simulink model "Battery_Connected_3_Phase_GridTied_Inverter"  (R2022a)
settings: Solver=ode3  StartTime=0.0  StopTime=4  FixedStep=dtsim  RelTol=1e-3
values from neighbouring files (symbols this model uses):
  a1_lpf = 1.3601/wc_lpf    (= 4.32933276199e-05)    [Battery_Connected_3_Phase_GridTied_Inverter_Parameters.m]    (also in NonDispDGParameters.m)
  a2_lpf = 0.6165/wc_lpf2    (= 6.24645097155e-10)    [Battery_Connected_3_Phase_GridTied_Inverter_Parameters.m]    (also in NonDispDGParameters.m)
  bf = 2 * eta * wc    [Battery_Connected_3_Phase_GridTied_Inverter_Parameters.m]    (also in NonDispDGParameters.m)
  C_HV = 100e-6    (= 0.0001)    [Battery_Connected_3_Phase_GridTied_Inverter_Parameters.m]    (also in NonDispDGParameters.m; power_converters_DAB_1ph_Parameters.m)
  C_LV = 2000e-6    (= 0.002)    [Battery_Connected_3_Phase_GridTied_Inverter_Parameters.m]    (also in NonDispDGParameters.m; power_converters_DAB_1ph_Parameters.m)
  Cdc = 2 * E_Cdc / Vdc / Vdc    (= 0.00125)    [Battery_Connected_3_Phase_GridTied_Inverter_Parameters.m]    (also in NonDispDGParameters.m)
  Cf = x*Cb    (= 7.95774715459e-06)    [Battery_Connected_3_Phase_GridTied_Inverter_Parameters.m]    (also in NonDispDGParameters.m = 8.72536076817e-06)
  cf = wc * wc    (= 15791.3670417)    [Battery_Connected_3_Phase_GridTied_Inverter_Parameters.m]    (also in NonDispDGParameters.m)
  Cs_FET = inf    [Battery_Connected_3_Phase_GridTied_Inverter_Parameters.m]    (also in NonDispDGParameters.m; power_converters_DAB_1ph_Parameters.m)
  dP1 = 0.3    [Battery_Connected_3_Phase_GridTied_Inverter_Parameters.m]    (also in NonDispDGParameters.m)
  dP2 = 0.5    [Battery_Connected_3_Phase_GridTied_Inverter_Parameters.m]    (also in NonDispDGParameters.m)
  dP3 = 0.8    [Battery_Connected_3_Phase_GridTied_Inverter_Parameters.m]    (also in NonDispDGParameters.m = 0.2)
  dP4 = -0.6    [Battery_Connected_3_Phase_GridTied_Inverter_Parameters.m]    (also in NonDispDGParameters.m)
  dtsim = 5.0e-6    (= 5e-06)    [Battery_Connected_3_Phase_GridTied_Inverter_Parameters.m]    (also in NonDispDGParameters.m)
  f0 = 50    [Battery_Connected_3_Phase_GridTied_Inverter_Parameters.m]    (also in NonDispDGParameters.m)
  Fsw = 10e3    (= 10000)    [Battery_Connected_3_Phase_GridTied_Inverter_Parameters.m]    (also in NonDispDGParameters.m; power_converters_DAB_1ph_Parameters.m = 5000)
  Ia_limit = 1    [Battery_Connected_3_Phase_GridTied_Inverter_Parameters.m]    (also in NonDispDGParameters.m)
  Ib_peak = Ib*sqrt(2)    [Battery_Connected_3_Phase_GridTied_Inverter_Parameters.m]    (also in NonDispDGParameters.m)
  Ir_limit = 1    [Battery_Connected_3_Phase_GridTied_Inverter_Parameters.m]    (also in NonDispDGParameters.m)
  Ki = Kp/Ti    [Battery_Connected_3_Phase_GridTied_Inverter_Parameters.m]    (also in NonDispDGParameters.m)
  Kii = (BW_conv/w0) * Rseries_pu * w0    [Battery_Connected_3_Phase_GridTied_Inverter_Parameters.m]    (also in NonDispDGParameters.m)
  Kip = BW_P    [Battery_Connected_3_Phase_GridTied_Inverter_Parameters.m]    (also in NonDispDGParameters.m)
  Kiq = BW_Q    [Battery_Connected_3_Phase_GridTied_Inverter_Parameters.m]    (also in NonDispDGParameters.m)
  Kp = 2/A0 * KP    [Battery_Connected_3_Phase_GridTied_Inverter_Parameters.m]    (also in NonDispDGParameters.m)
  Kpi = (BW_conv/w0) * Lseries_pu    [Battery_Connected_3_Phase_GridTied_Inverter_Parameters.m]    (also in NonDispDGParameters.m)
  Kpp = BW_P * Tconv    [Battery_Connected_3_Phase_GridTied_Inverter_Parameters.m]    (also in NonDispDGParameters.m)
  Kpq = BW_Q * Tconv    [Battery_Connected_3_Phase_GridTied_Inverter_Parameters.m]    (also in NonDispDGParameters.m)
  L_Inductor = 1000e-6    (= 0.001)    [Battery_Connected_3_Phase_GridTied_Inverter_Parameters.m]    (also in NonDispDGParameters.m; power_converters_DAB_1ph_Parameters.m = 8e-06)
  Lgrid = Xgrid/w0    (= 0.00795774715459)    [Battery_Connected_3_Phase_GridTied_Inverter_Parameters.m]    (also in NonDispDGParameters.m)
  Li = Vdc/(16*fsw*delta_Ilmax)    [Battery_Connected_3_Phase_GridTied_Inverter_Parameters.m]    (also in NonDispDGParameters.m)
  Li_pu = Li/Lb    [Battery_Connected_3_Phase_GridTied_Inverter_Parameters.m]    (also in NonDispDGParameters.m)
  Lm_Tr = 100e-3    (= 0.1)    [Battery_Connected_3_Phase_GridTied_Inverter_Parameters.m]    (also in NonDispDGParameters.m; power_converters_DAB_1ph_Parameters.m = 0.00072)
  Lprim_Tr = 1e-7    (= 1e-07)    [Battery_Connected_3_Phase_GridTied_Inverter_Parameters.m]    (also in NonDispDGParameters.m; power_converters_DAB_1ph_Parameters.m = 0)
  Lsec_Tr = 1e-7    (= 1e-07)    [Battery_Connected_3_Phase_GridTied_Inverter_Parameters.m]    (also in NonDispDGParameters.m; power_converters_DAB_1ph_Parameters.m = 1.7e-05)
  ma = E_ltl*sqrt(2)/Vdc    [Battery_Connected_3_Phase_GridTied_Inverter_Parameters.m]    (also in NonDispDGParameters.m)
  Ntran = Vmv/Vlv    (= 1.9)    [Battery_Connected_3_Phase_GridTied_Inverter_Parameters.m]    (also in NonDispDGParameters.m = 1.98952879581)
  phia = 0    [Battery_Connected_3_Phase_GridTied_Inverter_Parameters.m]    (also in NonDispDGParameters.m)
  Pinit = 0    [Battery_Connected_3_Phase_GridTied_Inverter_Parameters.m]    (also in NonDispDGParameters.m)
  Pnom = 1000    [Battery_Connected_3_Phase_GridTied_Inverter_Parameters.m]    (also in NonDispDGParameters.m; power_converters_DAB_1ph_Parameters.m = 10000)
  R_DCsrc1 = 1e-7    (= 1e-07)    [Battery_Connected_3_Phase_GridTied_Inverter_Parameters.m]    (also in NonDispDGParameters.m; power_converters_DAB_1ph_Parameters.m)
  R_Inductor = 16e-3    (= 0.016)    [Battery_Connected_3_Phase_GridTied_Inverter_Parameters.m]    (also in NonDispDGParameters.m; power_converters_DAB_1ph_Parameters.m)
  RC_HV = 1e-3    (= 0.001)    [Battery_Connected_3_Phase_GridTied_Inverter_Parameters.m]    (also in NonDispDGParameters.m; power_converters_DAB_1ph_Parameters.m)
  RC_LV = 1e-3    (= 0.001)    [Battery_Connected_3_Phase_GridTied_Inverter_Parameters.m]    (also in NonDispDGParameters.m; power_converters_DAB_1ph_Parameters.m)
  Rd = 1/(3*wres*Cf)    [Battery_Connected_3_Phase_GridTied_Inverter_Parameters.m]    (also in NonDispDGParameters.m)
  Rgrid = 0.7    [Battery_Connected_3_Phase_GridTied_Inverter_Parameters.m]    (also in NonDispDGParameters.m)
  Ri = Ri_pu*Zb    [Battery_Connected_3_Phase_GridTied_Inverter_Parameters.m]    (also in NonDispDGParameters.m)
  Rm_Tr = 1e6    (= 1000000)    [Battery_Connected_3_Phase_GridTied_Inverter_Parameters.m]    (also in NonDispDGParameters.m; power_converters_DAB_1ph_Parameters.m = 10000)
  Ron_Diode = 10e-3    (= 0.01)    [Battery_Connected_3_Phase_GridTied_Inverter_Parameters.m]    (also in NonDispDGParameters.m; power_converters_DAB_1ph_Parameters.m)
  Ron_FET = 20e-3    (= 0.02)    [Battery_Connected_3_Phase_GridTied_Inverter_Parameters.m]    (also in NonDispDGParameters.m; power_converters_DAB_1ph_Parameters.m = 0.016)
  Rprim_Tr = 10e-3    (= 0.01)    [Battery_Connected_3_Phase_GridTied_Inverter_Parameters.m]    (also in NonDispDGParameters.m; power_converters_DAB_1ph_Parameters.m = 1e-06)
  Rs_FET = 1e6    (= 1000000)    [Battery_Connected_3_Phase_GridTied_Inverter_Parameters.m]    (also in NonDispDGParameters.m; power_converters_DAB_1ph_Parameters.m)
  Rsec_Tr = 10e-3    (= 0.01)    [Battery_Connected_3_Phase_GridTied_Inverter_Parameters.m]    (also in NonDispDGParameters.m; power_converters_DAB_1ph_Parameters.m = 0.043)
  Rtran_pu = 0.003    [Battery_Connected_3_Phase_GridTied_Inverter_Parameters.m]    (also in NonDispDGParameters.m)
  Sb = Pinv    (= 1000)    [Battery_Connected_3_Phase_GridTied_Inverter_Parameters.m]    (also in NonDispDGParameters.m)
  Stran = 1000    [Battery_Connected_3_Phase_GridTied_Inverter_Parameters.m]    (also in NonDispDGParameters.m)
  tinit = 0.25    [Battery_Connected_3_Phase_GridTied_Inverter_Parameters.m]    (also in NonDispDGParameters.m)
  tP1 = 0.5    [Battery_Connected_3_Phase_GridTied_Inverter_Parameters.m]    (also in NonDispDGParameters.m)
  tP2 = 1.5    [Battery_Connected_3_Phase_GridTied_Inverter_Parameters.m]    (also in NonDispDGParameters.m)
  tP3 = 2.5    [Battery_Connected_3_Phase_GridTied_Inverter_Parameters.m]    (also in NonDispDGParameters.m)
  tP4 = 3.5    [Battery_Connected_3_Phase_GridTied_Inverter_Parameters.m]    (also in NonDispDGParameters.m)
  Ts = 1e-7    (= 1e-07)    [Battery_Connected_3_Phase_GridTied_Inverter_Parameters.m]    (also in NonDispDGParameters.m; power_converters_DAB_1ph_Parameters.m)
  Turn_ratio = 15    [Battery_Connected_3_Phase_GridTied_Inverter_Parameters.m]    (also in NonDispDGParameters.m; power_converters_DAB_1ph_Parameters.m)
  Vb_peak = Vb*sqrt(2/3)    [Battery_Connected_3_Phase_GridTied_Inverter_Parameters.m]    (also in NonDispDGParameters.m)
  Vbat = 25    [Battery_Connected_3_Phase_GridTied_Inverter_Parameters.m]    (also in NonDispDGParameters.m = 24; power_converters_DAB_1ph_Parameters.m = 24)
  Vc_prime = 0.25    [Battery_Connected_3_Phase_GridTied_Inverter_Parameters.m]    (also in NonDispDGParameters.m)
  Vdc = 400    [Battery_Connected_3_Phase_GridTied_Inverter_Parameters.m]    (also in NonDispDGParameters.m)
  Vf_Diode = 4.2    [Battery_Connected_3_Phase_GridTied_Inverter_Parameters.m]    (also in NonDispDGParameters.m; power_converters_DAB_1ph_Parameters.m)
  Vlv = 200    [Battery_Connected_3_Phase_GridTied_Inverter_Parameters.m]    (also in NonDispDGParameters.m = 191)
  Vmv = 380    [Battery_Connected_3_Phase_GridTied_Inverter_Parameters.m]    (also in NonDispDGParameters.m)
  w0 = 2*pi*f0    (= 314.159265359)    [Battery_Connected_3_Phase_GridTied_Inverter_Parameters.m]    (also in NonDispDGParameters.m)
  Xtran_pu = 0.6    [Battery_Connected_3_Phase_GridTied_Inverter_Parameters.m]    (also in NonDispDGParameters.m)
undefined symbols (not defined in the file or in its folder): D11, Delta, Ion, Lg, Lithium
libraries: spsDiodeLib x8, spsIdealSwitchLib x8, spsVoltageMeasurementLib x6, spsCurrentMeasurementLib x6, spsSeriesRLCBranchLib x5, slpidlib x5, simulink x3, spsControlledVoltageSourceLib x3, spsControlledCurrentSourceLib x2, simulink_extras x2, spsSawtoothGeneratorLib x2, spspowerguiLib x2
(part 1 of 2)
settings Model: Creator=Ulas  LastModifiedBy=Ethan
settings SolverCC: AlgebraicLoopSolver=TrustRegion
settings DataIOCC: ReturnWorkspaceOutputs=off
settings DebuggingCC: UnconnectedInputMsg=warning  UnconnectedOutputMsg=warning  UnconnectedLineMsg=warning  SFMachineParentedDataDiag=warning
settings SFSimCC: CustomCodeUndefinedFunction=UseInterfaceOnly
settings RTWCC: DLArmComputeVersion=19.05

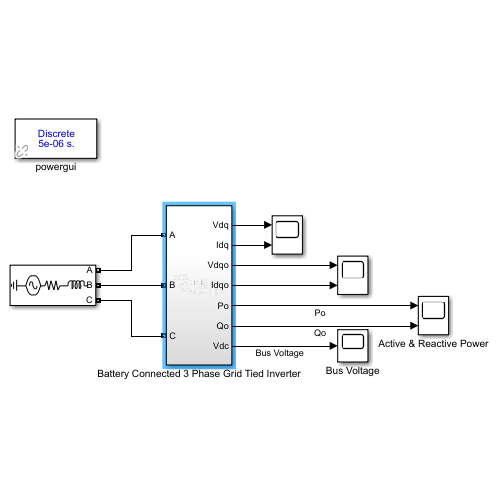
[thumbnail: Simulink's stored preview of the top-level diagram]
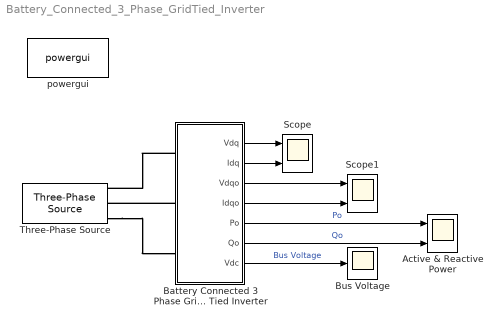
== system Battery_Connected_3_Phase_GridTied_Inverter ==
  Active & Reactive Power : Scope  NumInputPorts=2
  Battery Connected 3 Phase Grid Tied Inverter : Subsystem
  Bus Voltage : Scope
  Scope : Scope  NumInputPorts=2
  Scope1 : Scope  NumInputPorts=2
  Three-Phase Source : spsThreePhaseSourceLib/Three-Phase Source  InternalConnection=Yg  VoltagePhases=off  Voltage=Vmv  PhaseAngle=-30  Voltage_phases=[25e3 25e3 25e3]/sqrt(3)  PhaseAngles_phases=[0 -120 +120]  Frequency=f0  NonIdealSource=on  SpecifyImpedance=off  Resistance=Rgrid  Inductance=Lgrid  ShortCircuitLevel=100e6  BaseVoltage=Vmv  XRratio=7  BusType=swing  Pref=10e3  Qref=0  Prefabc=[10e3, 10e3, 10e3]  Qrefabc=[0, 0, 0]  Qmin=-inf  Qmax=inf
  powergui : spspowerguiLib/powergui  Priority=1  SimulationMode=Discrete  SampleTime=dtsim  frequency=60  Iterations=50  frequencyindice=0  Pbase=100e6  ErrMax=1e-4  UnitsV=kV  UnitsW=MW  buscounter=0  FunctionMessages=off  echomessages=off  EnableUseOfTLC=off  CurrentSourceSwitches=off  DisableSnubberDevices=off  DisableRonSwitches=off  DisableVfSwitches=off  DisplayEquations=off  AutomaticDiscreteSolvers=off  SolverType=Tustin/Backward Euler (TBE)  Interpol=off  ExternalGateDelay=off  methode=off  Ts=100  x0status=blocks  SPID=on  SwTol=0  HookPort=off  NonlinearTolerance=0  nMaxIteration=15  ContinueOnMaxIteration=off  RestoreLinks=warning  ResistiveCurrentMeasurement=off  Frange=[0:2:500]  Ylog=off  Xlog=on  ShowGrid=off  save=off  variable=ZData  structure=ScopeData  ZoomFFT=off  StartTime=0.5  cycles=5  DisplayStyle=1  fundamental=50  FreqAxis=off  MaxFrequency=1000  frequencyindicesteady=1  RmsSteady=2  display=off
  wires:
  Battery Connected 3 Phase Grid Tied Inverter/1(Vdq) -> Scope/1
  Battery Connected 3 Phase Grid Tied Inverter/2(Idq) -> Scope/2
  Battery Connected 3 Phase Grid Tied Inverter/3(Vdqo) -> Scope1/1
  Battery Connected 3 Phase Grid Tied Inverter/4(Idqo) -> Scope1/2
  Battery Connected 3 Phase Grid Tied Inverter/5(Po) -> Active & Reactive Power/1  "Po"
  Battery Connected 3 Phase Grid Tied Inverter/6(Qo) -> Active & Reactive Power/2  "Qo"
  Battery Connected 3 Phase Grid Tied Inverter/7(Vdc) -> Bus Voltage/1  "Bus Voltage"
  connections:
  Battery Connected 3 Phase Grid Tied Inverter/LConn2 -- Three-Phase Source/RConn2
  Battery Connected 3 Phase Grid Tied Inverter/LConn1 -- Three-Phase Source/RConn1
  Three-Phase Source/RConn3 -- Battery Connected 3 Phase Grid Tied Inverter/LConn3

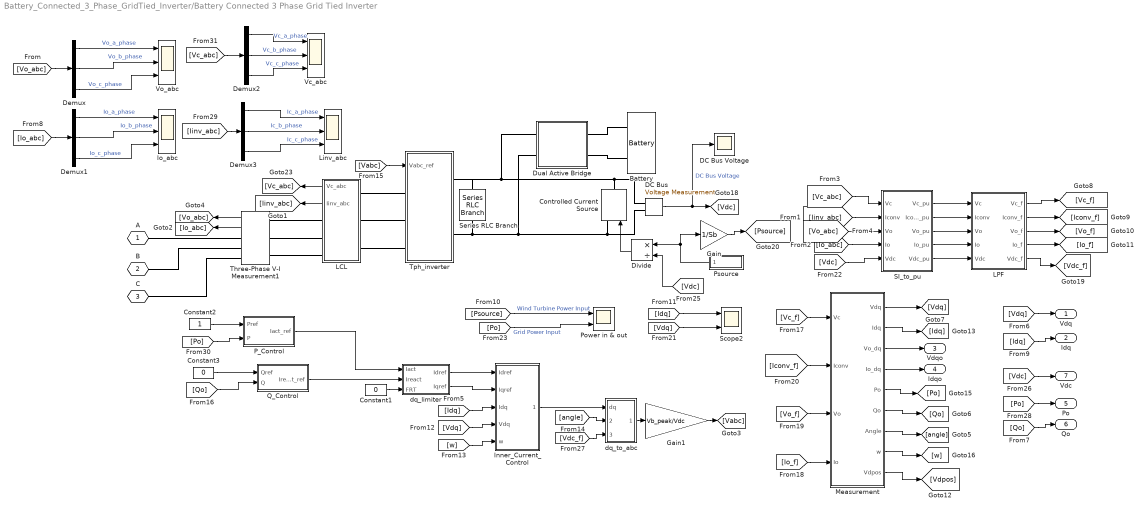
== system Battery_Connected_3_Phase_GridTied_Inverter/Battery Connected 3 Phase Grid Tied Inverter ==
  Battery : spsBatteryLib/Battery  BatType=Lithium-Ion  ShowTempParam=off  ThermalPreset=no  ShowAgeParam=off  NomV=24  NomQ=100  SOC=70  Batt_Tr=1  PresetModel=on  MaxQ=100  MinV=18  FullV=27.9357  Dis_rate=43.4783  R=0.0024  Normal_OP=90.4348  expZone="[25.9293      4.91304]"  current=[6.5 13 32.5]  Units=Time  Tci=20  NomT=20  T2=-30  MaxQ2=4.8  FullV2=7.1  Normal_OP2=5.655  expZone2="[6.58           1]"  Rca=0.6  ti=2000  Dp=0  Neq0=0  Tsim=1e6  Ta1=25  Qeol=5.4*0.9  Reol=0.013333*1.2  Char_age=[2.3478, 3]  Dis_age=[2.3478, 10]  N1=1500  N2=10500  N3=1000  N4=1400  Ta2=45  N5=950
  Constant1 : Constant  Value=0
  Constant2 : Constant
  Constant3 : Constant  Value=0
  Controlled Current Source : spsControlledCurrentSourceLib/Controlled Current Source  Initialize=on  Source_Type=AC  Amplitude=0  Phase=0  Frequency=0  Measurements=None
  DC Bus : spsVoltageMeasurementLib/Voltage Measurement  PhasorSimulation=off  OutputType=Complex  PSBequivalent=0
  DC Bus Voltage : Scope
  Demux{,1..3} (4 alike) : Demux  Outputs=3
  Divide : Product  Inputs=*/
  Dual Active Bridge : Subsystem
  Gain : Gain  Gain=1/Sb
  Gain1 : Gain  Gain=Vb_peak/Vdc
  Inner_Current_Control : Subsystem
  Io_abc : Scope  NumInputPorts=3
  LCL : Subsystem
  LPF : Subsystem
  Linv_abc : Scope  NumInputPorts=3
  Measurement : Subsystem
  P_Control : Subsystem
  Power in & out : Scope  NumInputPorts=2
  Psource : Subsystem
  Q_Control : Subsystem
  SI_to_pu : Subsystem
  Scope2 : Scope  NumInputPorts=2
  Series RLC Branch : spsSeriesRLCBranchLib/Series RLC Branch  LConnTagsString=__new0  RConnTagsString=__new0  BranchType=C  Resistance=1  Inductance=1e-3  SetiL0=off  InitialCurrent=0  Capacitance=Cdc  Setx0=on  InitialVoltage=Vdc  Measurements=None
  Three-Phase V-I Measurement1 : spsThreePhaseVIMeasurementLib/Three-Phase V-I Measurement  VoltageMeasurement=phase-to-ground  SetLabelV=off  LabelV=Vabc  Vpu=off  VpuLL=off  CurrentMeasurement=yes  SetLabelI=off  LabelI=Iabc  Ipu=off  Pbase=100e6  Vbase=500e3  OutputType=Complex  PhasorSimulation=off  PSBequivalent=0
  Tph_inverter : Subsystem
  Vc_abc : Scope  NumInputPorts=3
  Vo_abc : Scope  NumInputPorts=3
  dq_limiter : Subsystem
  dq_to_abc : Subsystem
  A : PMIOPort  Tag=PMCPort  Side=Left
  B : PMIOPort  Tag=PMCPort  Port=2  Side=Left
  C : PMIOPort  Tag=PMCPort  Port=3  Side=Left
  Vdq : Outport  VectorParamsAs1DForOutWhenUnconnected=off
  Idq : Outport  Port=2  VectorParamsAs1DForOutWhenUnconnected=off
  Vdqo : Outport  Port=3  VectorParamsAs1DForOutWhenUnconnected=off
  Idqo : Outport  Port=4  VectorParamsAs1DForOutWhenUnconnected=off
  Po : Outport  Port=5  VectorParamsAs1DForOutWhenUnconnected=off
  Qo : Outport  Port=6  VectorParamsAs1DForOutWhenUnconnected=off
  Vdc : Outport  Port=7  VectorParamsAs1DForOutWhenUnconnected=off
  wires:
  [Vabc] -> Tph_inverter/1(Vabc_ref)
  Three-Phase V-I Measurement1/1 -> [Vo_abc]
  LCL/1(Vc_abc) -> [Vc_abc]
  Three-Phase V-I Measurement1/2 -> [Io_abc]
  LCL/2(Iinv_abc) -> [Iinv_abc]
  Constant1/1 -> dq_limiter/3(FRT)
  [Vdc_f] -> dq_to_abc/3(Vdc)
  dq_limiter/1(Idref) -> Inner_Current_Control/1(Idref)
  Q_Control/1(Ireact_ref) -> dq_limiter/2(Ireact)
  dq_to_abc/1(abc) -> Gain1/1
  [Vdq] -> Inner_Current_Control/4(Vdq)
  Gain1/1 -> [Vabc]
  Inner_Current_Control/1(Vdq_ref) -> dq_to_abc/1(dq)
  [w] -> Inner_Current_Control/5(w)
  [angle] -> dq_to_abc/2(theta)
  [Qo] -> Q_Control/2(Q)
  [Idq] -> Inner_Current_Control/3(Idq)
  dq_limiter/2(Iqref) -> Inner_Current_Control/2(Iqref)
  [Vdc] -> SI_to_pu/5(Vdc)
  SI_to_pu/3(Vo_pu) -> LPF/3(Vo)
  LPF/5(Vdc_f) -> [Vdc_f]
  [Vc_abc] -> SI_to_pu/1(Vc)
  Measurement/9(Vdpos) -> [Vdpos]
  LPF/4(Io_f) -> [Io_f]
  LPF/2(Iconv_f) -> [Iconv_f]
  [Vo_abc] -> SI_to_pu/3(Vo)
  LPF/3(Vo_f) -> [Vo_f]
  Measurement/2(Idq) -> [Idq]
  Measurement/1(Vdq) -> [Vdq]
  [Vc_f] -> Measurement/1(Vc)
  [Vdq] -> Vdq/1
  [Io_f] -> Measurement/4(Io)
  SI_to_pu/5(Vdc_pu) -> LPF/5(Vdc)
  [Vo_f] -> Measurement/3(Vo)
  [Iconv_f] -> Measurement/2(Iconv)
  LPF/1(Vc_f) -> [Vc_f]
  Measurement/8(w) -> [w]
  [Iinv_abc] -> SI_to_pu/2(Iconv)
  Measurement/4(Io_dq) -> Idqo/1
  Measurement/7(Angle) -> [angle]
  SI_to_pu/4(Io_pu) -> LPF/4(Io)
  [Vdc] -> Vdc/1
  Measurement/3(Vo_dq) -> Vdqo/1
  [Idq] -> Idq/1
  SI_to_pu/1(Vc_pu) -> LPF/1(Vc)
  SI_to_pu/2(Iconv_pu) -> LPF/2(Iconv)
  [Io_abc] -> SI_to_pu/4(Io)
  [Qo] -> Qo/1
  Measurement/6(Qo) -> [Qo]
  [Idq] -> Scope2/1
  [Vdq] -> Scope2/2
  Divide/1 -> Controlled Current Source/1
  [Vdc] -> Divide/2
  Gain/1 -> [Psource]
  DC Bus/1 -> DC Bus Voltage/1, [Vdc]  "DC Bus Voltage"
  [Psource] -> Power in & out/1  "Wind Turbine Power Input"
  [Po] -> Power in & out/2  "Grid Power Input"
  Measurement/5(Po) -> [Po]
  [Po] -> Po/1
  Constant3/1 -> Q_Control/1(Qref)
  Psource/1(Psource) -> Divide/1, Gain/1
  Demux/2 -> Vo_abc/2  "Vo_b_phase"
  Demux/1 -> Vo_abc/1  "Vo_a_phase"
  Demux/3 -> Vo_abc/3  "Vo_c_phase"
  [Vo_abc] -> Demux/1
  Demux1/2 -> Io_abc/2  "Io_b_phase"
  Demux1/1 -> Io_abc/1  "Io_a_phase"
  Demux1/3 -> Io_abc/3  "Io_c_phase"
  [Io_abc] -> Demux1/1
  [Vc_abc] -> Demux2/1
  Demux2/2 -> Vc_abc/2  "Vc_b_phase"
  Demux2/1 -> Vc_abc/1  "Vc_a_phase"
  Demux2/3 -> Vc_abc/3  "Vc_c_phase"
  Demux3/3 -> Linv_abc/3  "Ic_c_phase"
  Demux3/2 -> Linv_abc/2  "Ic_b_phase"
  Demux3/1 -> Linv_abc/1  "Ic_a_phase"
  [Iinv_abc] -> Demux3/1
  P_Control/1(Iact_ref) -> dq_limiter/1(Iact)
  [Po] -> P_Control/2(P)
  Constant2/1 -> P_Control/1(Pref)
  connections:
  DC Bus/LConn1 -- Dual Active Bridge/LConn1 -- Tph_inverter/RConn1 -- Series RLC Branch/LConn1 -- Controlled Current Source/RConn1
  DC Bus/LConn2 -- Controlled Current Source/LConn1 -- Tph_inverter/RConn2 -- Series RLC Branch/RConn1 -- Dual Active Bridge/LConn2
  C/RConn1 -- Three-Phase V-I Measurement1/RConn3
  Tph_inverter/LConn2 -- LCL/LConn2
  Tph_inverter/LConn3 -- LCL/LConn3
  Three-Phase V-I Measurement1/LConn1 -- LCL/RConn1
  A/RConn1 -- Three-Phase V-I Measurement1/RConn1
  Tph_inverter/LConn1 -- LCL/LConn1
  B/RConn1 -- Three-Phase V-I Measurement1/RConn2
  Three-Phase V-I Measurement1/LConn2 -- LCL/RConn2
  Three-Phase V-I Measurement1/LConn3 -- LCL/RConn3
  Battery/LConn1 -- Dual Active Bridge/RConn1
  Battery/LConn2 -- Dual Active Bridge/RConn2

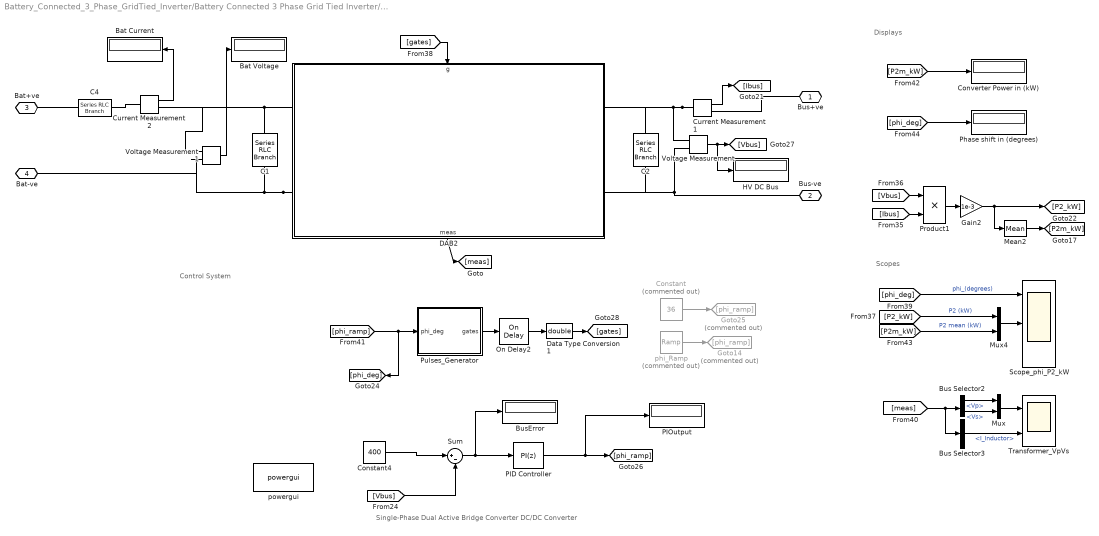
== system Battery_Connected_3_Phase_GridTied_Inverter/Battery Connected 3 Phase Grid Tied Inverter/Dual Active Bridge ==
  note: Control System
  note: Displays
  note: Scopes
  note: Single-Phase Dual Active Bridge Converter DC/DC Converter
  Bat Current : Display
      settings: Format=bank  Decimation=100
  Bat Voltage : Display
      settings: Format=bank  Decimation=100
  Bus Selector2 : BusSelector  OutputSignals=Vp,Vs
  Bus Selector3 : BusSelector  OutputSignals=I_Inductor
  BusError : Display
      settings: Format=bank  Decimation=100
  C1 : spsSeriesRLCBranchLib/Series RLC Branch  LConnTagsString=__new0  RConnTagsString=__new0  BranchType=RC  Resistance=RC_LV  Inductance=1  SetiL0=off  InitialCurrent=0  Capacitance=C_LV  Setx0=off  InitialVoltage=0  Measurements=None
  C2 : spsSeriesRLCBranchLib/Series RLC Branch  LConnTagsString=__new0  RConnTagsString=__new0  BranchType=RC  Resistance=RC_HV  Inductance=1  SetiL0=off  InitialCurrent=0  Capacitance=C_HV  Setx0=off  InitialVoltage=0  Measurements=None
  C4 : spsSeriesRLCBranchLib/Series RLC Branch  LConnTagsString=__new0  RConnTagsString=__new0  BranchType=R  Resistance=R_DCsrc1  Inductance=1  SetiL0=off  InitialCurrent=0  Capacitance=1  Setx0=off  InitialVoltage=0  Measurements=None
  Constant : Constant  Commented=on  Value=36
  Constant4 : Constant  Value=400
  Converter Power in (kW) : Display
      settings: Format=bank  Decimation=100
  Current Measurement1 : spsCurrentMeasurementLib/Current Measurement  PhasorSimulation=off  OutputType=Complex  PSBequivalent=0
  Current Measurement2 : spsCurrentMeasurementLib/Current Measurement  PhasorSimulation=off  OutputType=Complex  PSBequivalent=0
  DAB2 : Subsystem  mask(Single-phase, Dual-Active Bridge DC/DC Converter){Ron_FET=Ron_FET, RsCs_FET=[Rs_FET, Cs_FET], Ron_Diode=Ron_Diode, Vf_Diode=Vf_Diode, RL_Inductor=[R_Inductor, L_Inductor], Param1_Tr=[Pnom, Fsw], Param2_Tr=[Vbat, Rprim_Tr, Lprim_Tr], Param3_Tr=[Vbat*Turn_ratio, Rsec_Tr, Lsec_Tr], Param4_Tr=[Rm_Tr, Lm_Tr]}
      mask prompts: Ron_FET "Ron FET"; RsCs_FET "FET snubber: [Rs (ohm)  Cs (F)]"; RL_Inductor "Coupling inductor [ R (ohms)   L (H)]"; Param1_Tr "Nominal power and frequency [Pn(VA) fn(Hz)]:"; Param2_Tr "Winding 1 parameters [V1(Vrms) R1(ohm) L1(H)]:"; Param3_Tr "Winding 2 parameters [V2(Vrms) R2(ohm) L2(H)]:"; Param4_Tr "Magnetization resistance and inductance [Rm(ohm) Lm(H)]:"
      mask init:
      | Rs_FET=RsCs_FET(1);
      | Cs_FET=RsCs_FET(2);
      | R_Inductor=RL_Inductor(1);
      | L_Inductor=RL_Inductor(2);
      settings: PortSchema="{\"entries\":[{\"content\":{\"sides\":[{\"content\":{\"connectorIds\":[\"LConn1\",\"LConn2\"]},\"type\":\"ConnectorPlacement.EquallySpacedRectSide\",\"uuid\":\"9324ea44-499c-4ecb-9e49-362befe9c555\"},{\"content\":{\"connectorIds\":[\"RConn1\",\"RConn2\"],\"side\":\"RIGHT\"},\"type\":\"ConnectorPlacement.EquallySpacedRectSide\",\"uuid\":\"1d2d188e-4a2f-457a-9d2e-cac68811a3aa\"},{\"content\":{\"connectorIds\":[\"In1\"],\"side\":\"TOP\"},\"type\":\"ConnectorPlacement.EquallySpacedRectSide\",\"uuid\":\"7f41b21e-a624-46b0-bf38-abdafc8e74d0\"},{\"content\":{\"connectorIds\":[\"Out1\"],\"side\":\"BOTTOM\"},\"type\":\"ConnectorPlacement.EquallySpacedRectSide\",\"uuid\":\"ef27d855-3875-49de-80dc-d9576eabadca\"}]},\"type\":\"ConnectorPlacement.EquallySpacedConnector\",\"uuid\":\"30393c4b-568d-4140-9cdd-d3267fa7bc9d\"}],\"packageUris\":[\"http://schema.mathworks.com/mf0/Connector/R2020b\"],\"version\":\"1.0\"}"
      mask Display: image('DAB_FB1.png')
  Data Type Conversion1 : DataTypeConversion  OutDataTypeStr=double  SaturateOnIntegerOverflow=off  RndMeth=Floor
  Gain2 : Gain  Gain=1e-3
  Goto14 : Goto  Commented=on  GotoTag=phi_ramp
  Goto25 : Goto  Commented=on  GotoTag=phi_ramp
  HV DC Bus : Display
      settings: Format=bank  Decimation=100
  Mean2 : spsMeanLib/Mean  Freq=Fsw  Vinit=0  Ts=0
  Mux : Mux  Inputs=2
  Mux4 : Mux  Inputs=2
  On Delay2 : spsOnDelayLib/On Delay  DelayType=On delay  delay=DT  ic=0  Ts=0
      settings: SourceProductBaseCode=PS
  PID Controller : slpidlib/PID Controller  Controller=PI  Form=Parallel  TimeDomain=Discrete-time  UseExternalTs=off  SampleTime=-1  IntegratorMethod=Forward Euler  FilterMethod=Forward Euler  ControllerParametersSource=internal  P=0.3  I=11  UseKiTs=off  D=0  N=100  UseFilter=on  TunerSelectOption=Transfer Function Based (PID Tuner App)  ZeroCross=off  InitialConditionSource=internal  InitialConditionForIntegrator=0  InitialConditionForFilter=0  DifferentiatorICPrevScaledInput=0  ExternalReset=none  TrackingMode=off  Kt=1  LimitOutput=off  SatLimitsSource=internal  UpperSaturationLimit=inf  LowerSaturationLimit=-inf  LinearizeAsGain=on  AntiWindupMode=none  Kb=1  POutMin=[]  POutMax=[]  IOutMin=[]  IOutMax=[]  DOutMin=[]  DOutMax=[]  NOutMin=[]  NOutMax=[]  SumOutMin=[]  SumOutMax=[]  SaturationOutMin=[]  SaturationOutMax=[]  PParamMin=[]  PParamMax=[]  IParamMin=[]  IParamMax=[]  DParamMin=[]  DParamMax=[]  NParamMin=[]  NParamMax=[]  KbParamMin=[]  KbParamMax=[]  KtParamMin=[]  KtParamMax=[]  KbOutMin=[]  KbOutMax=[]  KtOutMin=[]  KtOutMax=[]  IntegratorOutMin=[]  IntegratorOutMax=[]  FilterOutMin=[]  FilterOutMax=[]  SumI1OutMin=[]  SumI1OutMax=[]  SumI2OutMin=[]  SumI2OutMax=[]  SumI3OutMin=[]  SumI3OutMax=[]  SumI4OutMin=[]  SumI4OutMax=[]  SumDOutMin=[]  SumDOutMax=[]  DifferentiatorOutMin=[]  DifferentiatorOutMax=[]  FilterDiffOutCoefMin=[]  FilterDiffOutCoefMax=[]  ReciprocalOutMin=[]  ReciprocalOutMax=[]  SumDenOutMin=[]  SumDenOutMax=[]  SumNumOutMin=[]  SumNumOutMax=[]  DivideOutMin=[]  DivideOutMax=[]  UdiffTsProdOutMin=[]  UdiffTsProdOutMax=[]  NTsProdOutMin=[]  NTsProdOutMax=[]  UintegralTsProdOutMin=[]  UintegralTsProdOutMax=[]  UngainTsProdOutMin=[]  UngainTsProdOutMax=[]  IntegratorContinuousStateAttributes=''  IntegratorStateMustResolveToSignalObject=off  IntegratorRTWStateStorageClass=Auto  FilterContinuousStateAttributes=''  FilterStateMustResolveToSignalObject=off  FilterRTWStateStorageClass=Auto  ParallelPVariant=InternalParameters  IdealPVariant=Disabled  IVariant=InternalParameters  DVariant=Disabled  IntegratorVariant=Discrete  SatVariant=Disabled  AWVariant=Passthrough  PCopyVariant=Disabled  TRVariant=Disabled  FdbkBlocksVariant=Forward  IdealPFdbkVariant=Disabled  SatFdbkVariant=Disabled  DerivativeFilterVariant=Disabled  NVariant=Disabled  NCopyVariant=Disabled_SignalSpec  FilterICVariant=Disabled  IntegratorICVariant=InternalICs  ExternalResetVariant=Disabled  TRSumVariant=Passthrough  SumFdbkVariant=Disabled  SumVariant=Sum_PI  TsampFilterVariant=InternalTs  TsampNgainVariant=Passthrough  TsampIntegralVariant=Passthrough  ExternalSaturationOutDataTypeStr=Inherit: Same as second input  aMode=0
  PIOutput : Display
      settings: Format=bank  Decimation=100
  Phase shift in (degrees) : Display
      settings: Format=bank  Decimation=100
  Product1 : Product
  Pulses_Generator : Subsystem
  Scope_phi_P2_kW : Scope  NumInputPorts=3
  Sum : Sum  Inputs=|+-
  Transformer_VpVs : Scope  NumInputPorts=2
  Voltage Measurement : spsVoltageMeasurementLib/Voltage Measurement  PhasorSimulation=off  OutputType=Complex  PSBequivalent=0
  Voltage Measurement1 : spsVoltageMeasurementLib/Voltage Measurement  PhasorSimulation=off  OutputType=Complex  PSBequivalent=0
  phi_Ramp : simulink/Sources/Ramp  Commented=on  slope=200*1/0.04  start=0  InitialOutput=-100
  powergui : spspowerguiLib/powergui  Priority=1  SimulationMode=Discrete  SampleTime=Ts  frequency=60  Iterations=50  frequencyindice=0  Pbase=100e6  ErrMax=1e-4  UnitsV=kV  UnitsW=MW  buscounter=0  FunctionMessages=off  echomessages=off  EnableUseOfTLC=off  CurrentSourceSwitches=on  DisableSnubberDevices=off  DisableRonSwitches=off  DisableVfSwitches=off  DisplayEquations=off  AutomaticDiscreteSolvers=off  SolverType=Tustin/Backward Euler (TBE)  Interpol=off  ExternalGateDelay=off  methode=off  Ts=10  x0status=blocks  SPID=on  SwTol=0  HookPort=off  NonlinearTolerance=1e-4  nMaxIteration=100  ContinueOnMaxIteration=off  RestoreLinks=warning  ResistiveCurrentMeasurement=off  Frange=[0:2:500]  Ylog=off  Xlog=on  ShowGrid=off  save=off  variable=ZData  structure=0  ZoomFFT=off  StartTime=0.0  cycles=1  DisplayStyle=1  fundamental=60  FreqAxis=off  MaxFrequency=1000  frequencyindicesteady=1  RmsSteady=1  display=off
  Bus+ve : PMIOPort  Side=Left
  Bus-ve : PMIOPort  Port=2  Side=Left
  Bat+ve : PMIOPort  Port=3  Side=Right
  Bat-ve : PMIOPort  Port=4  Side=Right
  wires:
  [P2_kW] -> Mux4/1  "P2 (kW)"
  Bus Selector3/1 -> Transformer_VpVs/2  "<I_Inductor>"
  On Delay2/1 -> Data Type Conversion1/1
  [P2m_kW] -> Converter Power in (kW)/1
  phi_Ramp/1 -> Goto14/1
  [phi_deg] -> Phase shift in (degrees)/1
  Constant4/1 -> Sum/1
  Bus Selector2/1 -> Mux/1  "<Vp>"
  Mux/1 -> Transformer_VpVs/1
  [phi_ramp] -> [phi_deg], Pulses_Generator/1(phi_deg)
  Bus Selector2/2 -> Mux/2  "<Vs>"
  Mux4/1 -> Scope_phi_P2_kW/2
  Voltage Measurement1/1 -> Bat Voltage/1
  PID Controller/1 -> PIOutput/1, [phi_ramp]
  [Vbus] -> Sum/2
  Gain2/1 -> Mean2/1, [P2_kW]
  Sum/1 -> BusError/1, PID Controller/1
  Current Measurement1/1 -> [Ibus]
  [meas] -> Bus Selector3/1, Bus Selector2/1
  [P2m_kW] -> Mux4/2  "P2 mean (kW)"
  [Vbus] -> Product1/1
  Voltage Measurement/1 -> HV DC Bus/1, [Vbus]
  Constant/1 -> Goto25/1
  Data Type Conversion1/1 -> [gates]
  Pulses_Generator/1(gates) -> On Delay2/1
  [Ibus] -> Product1/2
  Mean2/1 -> [P2m_kW]
  [phi_deg] -> Scope_phi_P2_kW/1  "phi_(degrees)"
  [gates] -> DAB2/1(g)
  DAB2/1(meas) -> [meas]
  Product1/1 -> Gain2/1
  Current Measurement2/1 -> Bat Current/1
  connections:
  DAB2/LConn2 -- Bat-ve/RConn1 -- Voltage Measurement1/LConn2 -- C1/LConn1
  Voltage Measurement/LConn2 -- DAB2/RConn2 -- C2/LConn1 -- Bus-ve/RConn1
  Current Measurement1/LConn1 -- C2/RConn1 -- DAB2/RConn1 -- Voltage Measurement/LConn1
  C1/RConn1 -- Current Measurement2/RConn1 -- Voltage Measurement1/LConn1 -- DAB2/LConn1
  Bus+ve/RConn1 -- Current Measurement1/RConn1
  C4/RConn1 -- Bat+ve/RConn1
  Current Measurement2/LConn1 -- C4/LConn1

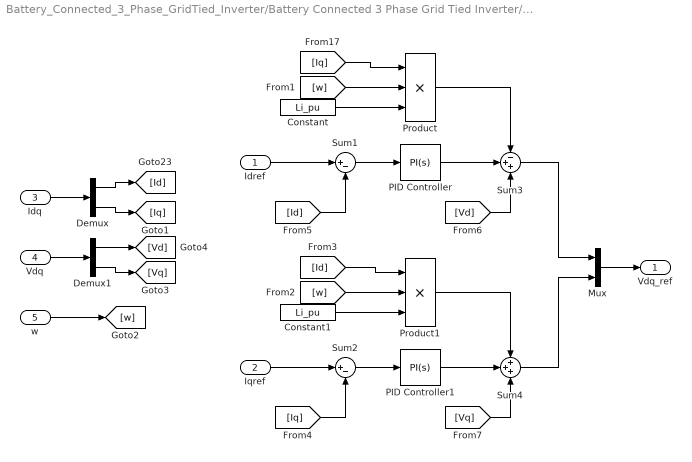
== system Battery_Connected_3_Phase_GridTied_Inverter/Battery Connected 3 Phase Grid Tied Inverter/Inner_Current_Control ==
  Idref : Inport
  Iqref : Inport  Port=2
  Idq : Inport  Port=3
  Vdq : Inport  Port=4
  w : Inport  Port=5
  Constant : Constant  Value=Li_pu
  Constant1 : Constant  Value=Li_pu
  Demux : Demux  Outputs=2
  Demux1 : Demux  Outputs=2
  Mux : Mux  Inputs=2
  PID Controller : slpidlib/PID Controller  Controller=PI  Form=Parallel  TimeDomain=Continuous-time  UseExternalTs=off  SampleTime=-1  IntegratorMethod=Forward Euler  FilterMethod=Forward Euler  ControllerParametersSource=internal  P=Kpi  I=Kii  UseKiTs=off  D=0  N=100  UseFilter=on  TunerSelectOption=Transfer Function Based (PID Tuner App)  InitialConditionSource=internal  InitialConditionForIntegrator=0  InitialConditionForFilter=0  DifferentiatorICPrevScaledInput=0  ExternalReset=none  TrackingMode=off  Kt=1  LimitOutput=on  SatLimitsSource=internal  UpperSaturationLimit=Vc_prime  LowerSaturationLimit=-Vc_prime  LinearizeAsGain=on  AntiWindupMode=clamping  Kb=1  POutMin=[]  POutMax=[]  IOutMin=[]  IOutMax=[]  DOutMin=[]  DOutMax=[]  NOutMin=[]  NOutMax=[]  SumOutMin=[]  SumOutMax=[]  SaturationOutMin=[]  SaturationOutMax=[]  PParamMin=[]  PParamMax=[]  IParamMin=[]  IParamMax=[]  DParamMin=[]  DParamMax=[]  NParamMin=[]  NParamMax=[]  KbParamMin=[]  KbParamMax=[]  KtParamMin=[]  KtParamMax=[]  KbOutMin=[]  KbOutMax=[]  KtOutMin=[]  KtOutMax=[]  IntegratorOutMin=[]  IntegratorOutMax=[]  FilterOutMin=[]  FilterOutMax=[]  SumI1OutMin=[]  SumI1OutMax=[]  SumI2OutMin=[]  SumI2OutMax=[]  SumI3OutMin=[]  SumI3OutMax=[]  SumI4OutMin=[]  SumI4OutMax=[]  SumDOutMin=[]  SumDOutMax=[]  DifferentiatorOutMin=[]  DifferentiatorOutMax=[]  FilterDiffOutCoefMin=[]  FilterDiffOutCoefMax=[]  ReciprocalOutMin=[]  ReciprocalOutMax=[]  SumDenOutMin=[]  SumDenOutMax=[]  SumNumOutMin=[]  SumNumOutMax=[]  DivideOutMin=[]  DivideOutMax=[]  UdiffTsProdOutMin=[]  UdiffTsProdOutMax=[]  NTsProdOutMin=[]  NTsProdOutMax=[]  UintegralTsProdOutMin=[]  UintegralTsProdOutMax=[]  UngainTsProdOutMin=[]  UngainTsProdOutMax=[]  IntegratorContinuousStateAttributes=''  IntegratorStateMustResolveToSignalObject=off  IntegratorRTWStateStorageClass=Auto  FilterContinuousStateAttributes=''  FilterStateMustResolveToSignalObject=off  FilterRTWStateStorageClass=Auto  ParallelPVariant=InternalParameters  IdealPVariant=Disabled  IVariant=InternalParameters  DVariant=Disabled  IntegratorVariant=Continuous  SatVariant=Enabled  AWVariant=ContClampingParallel  PCopyVariant=Disabled  TRVariant=Disabled  FdbkBlocksVariant=Forward  IdealPFdbkVariant=Disabled  SatFdbkVariant=Disabled  DerivativeFilterVariant=Disabled  NVariant=Disabled  NCopyVariant=Disabled_SignalSpec  FilterICVariant=Disabled  IntegratorICVariant=InternalICs  ExternalResetVariant=Disabled  TRSumVariant=Passthrough  SumFdbkVariant=Disabled  SumVariant=Sum_PI  TsampFilterVariant=InternalTs  TsampNgainVariant=Passthrough  TsampIntegralVariant=Passthrough  ExternalSaturationOutDataTypeStr=Inherit: Same as second input  aMode=0
  PID Controller1 : slpidlib/PID Controller  Controller=PI  Form=Parallel  TimeDomain=Continuous-time  UseExternalTs=off  SampleTime=-1  IntegratorMethod=Forward Euler  FilterMethod=Forward Euler  ControllerParametersSource=internal  P=Kpi  I=Kii  UseKiTs=off  D=0  N=100  UseFilter=on  TunerSelectOption=Transfer Function Based (PID Tuner App)  InitialConditionSource=internal  InitialConditionForIntegrator=0  InitialConditionForFilter=0  DifferentiatorICPrevScaledInput=0  ExternalReset=none  TrackingMode=off  Kt=1  LimitOutput=on  SatLimitsSource=internal  UpperSaturationLimit=Vc_prime  LowerSaturationLimit=-Vc_prime  LinearizeAsGain=on  AntiWindupMode=clamping  Kb=1  POutMin=[]  POutMax=[]  IOutMin=[]  IOutMax=[]  DOutMin=[]  DOutMax=[]  NOutMin=[]  NOutMax=[]  SumOutMin=[]  SumOutMax=[]  SaturationOutMin=[]  SaturationOutMax=[]  PParamMin=[]  PParamMax=[]  IParamMin=[]  IParamMax=[]  DParamMin=[]  DParamMax=[]  NParamMin=[]  NParamMax=[]  KbParamMin=[]  KbParamMax=[]  KtParamMin=[]  KtParamMax=[]  KbOutMin=[]  KbOutMax=[]  KtOutMin=[]  KtOutMax=[]  IntegratorOutMin=[]  IntegratorOutMax=[]  FilterOutMin=[]  FilterOutMax=[]  SumI1OutMin=[]  SumI1OutMax=[]  SumI2OutMin=[]  SumI2OutMax=[]  SumI3OutMin=[]  SumI3OutMax=[]  SumI4OutMin=[]  SumI4OutMax=[]  SumDOutMin=[]  SumDOutMax=[]  DifferentiatorOutMin=[]  DifferentiatorOutMax=[]  FilterDiffOutCoefMin=[]  FilterDiffOutCoefMax=[]  ReciprocalOutMin=[]  ReciprocalOutMax=[]  SumDenOutMin=[]  SumDenOutMax=[]  SumNumOutMin=[]  SumNumOutMax=[]  DivideOutMin=[]  DivideOutMax=[]  UdiffTsProdOutMin=[]  UdiffTsProdOutMax=[]  NTsProdOutMin=[]  NTsProdOutMax=[]  UintegralTsProdOutMin=[]  UintegralTsProdOutMax=[]  UngainTsProdOutMin=[]  UngainTsProdOutMax=[]  IntegratorContinuousStateAttributes=''  IntegratorStateMustResolveToSignalObject=off  IntegratorRTWStateStorageClass=Auto  FilterContinuousStateAttributes=''  FilterStateMustResolveToSignalObject=off  FilterRTWStateStorageClass=Auto  ParallelPVariant=InternalParameters  IdealPVariant=Disabled  IVariant=InternalParameters  DVariant=Disabled  IntegratorVariant=Continuous  SatVariant=Enabled  AWVariant=ContClampingParallel  PCopyVariant=Disabled  TRVariant=Disabled  FdbkBlocksVariant=Forward  IdealPFdbkVariant=Disabled  SatFdbkVariant=Disabled  DerivativeFilterVariant=Disabled  NVariant=Disabled  NCopyVariant=Disabled_SignalSpec  FilterICVariant=Disabled  IntegratorICVariant=InternalICs  ExternalResetVariant=Disabled  TRSumVariant=Passthrough  SumFdbkVariant=Disabled  SumVariant=Sum_PI  TsampFilterVariant=InternalTs  TsampNgainVariant=Passthrough  TsampIntegralVariant=Passthrough  ExternalSaturationOutDataTypeStr=Inherit: Same as second input  aMode=0
  Product : Product  Inputs=3
  Product1 : Product  Inputs=3
  Sum1 : Sum  Inputs=|+-
  Sum2 : Sum  Inputs=|+-
  Sum3 : Sum  Inputs=-++
  Sum4 : Sum  Inputs=+++
  Vdq_ref : Outport  VectorParamsAs1DForOutWhenUnconnected=off
  wires:
  Idref/1 -> Sum1/1
  [Iq] -> Sum2/2
  [Id] -> Sum1/2
  Iqref/1 -> Sum2/1
  [Iq] -> Product/1
  [w] -> Product/2
  Constant/1 -> Product/3
  [Id] -> Product1/1
  [w] -> Product1/2
  Constant1/1 -> Product1/3
  [Vq] -> Sum4/3
  PID Controller/1 -> Sum3/2
  PID Controller1/1 -> Sum4/2
  Idq/1 -> Demux/1
  Vdq/1 -> Demux1/1
  Demux/1 -> [Id]
  Demux/2 -> [Iq]
  Demux1/1 -> [Vd]
  Demux1/2 -> [Vq]
  w/1 -> [w]
  [Vd] -> Sum3/3
  Sum2/1 -> PID Controller1/1
  Sum1/1 -> PID Controller/1
  Sum3/1 -> Mux/1
  Sum4/1 -> Mux/2
  Mux/1 -> Vdq_ref/1
  Product1/1 -> Sum4/1
  Product/1 -> Sum3/1

== system Battery_Connected_3_Phase_GridTied_Inverter/Battery Connected 3 Phase Grid Tied Inverter/LCL ==
  Ground : spsGroundLib/Ground  LConnTagsString=a
  Li : spsThreePhaseSeriesRLCBranchLib/Three-Phase Series RLC Branch  LConnTagsString=A|B|C  RConnTagsString=A|B|C  BranchType=RL  Resistance=Ri  Inductance=Li  Capacitance=1e-6  Measurements=None
  Three-Phase Series RLC Branch2 : spsThreePhaseSeriesRLCBranchLib/Three-Phase Series RLC Branch  LConnTagsString=A|B|C  RConnTagsString=A|B|C  BranchType=RC  Resistance=Rd  Inductance=Lg  Capacitance=Cf  Measurements=None
  Three-Phase Transformer (Two Windings) : spsThreePhaseTransformerTwoWindingsLib/Three-Phase Transformer (Two Windings)  Winding1Connection=Delta (D11)  Winding2Connection=Yg  CoreType=Three single-phase transformers  SetSaturation=off  Hysteresis=off  DataFile='hysteresis'  SetInitialFlux=off  Measurements=None  UNITS=pu  NominalPower=[ Stran , f0 ]  Winding1=[Vmv , Rtran_pu/2 , Xtran_pu/2]  Winding2=[Vlv , Rtran_pu/2 , Xtran_pu/2]  Rm=500  Lm=500  L0=0.5  Saturation=[ 0,0 ; 0.0024,1.2 ; 1.0,1.52 ]  InitialFluxes=[ 0.8 , -0.8 , 0.7 ]  BreakLoop=off  DiscreteSolver=Trapezoidal iterative  DataType=off  TransfoNumber=1
  Three-Phase V-I Measurement : spsThreePhaseVIMeasurementLib/Three-Phase V-I Measurement  VoltageMeasurement=phase-to-ground  SetLabelV=off  LabelV=Vabc  Vpu=off  VpuLL=off  CurrentMeasurement=yes  SetLabelI=off  LabelI=Iabc  Ipu=off  Pbase=100e6  Vbase=500e3  OutputType=Complex  PhasorSimulation=off  PSBequivalent=0
  a : PMIOPort  Side=Right
  b : PMIOPort  Port=2  Side=Right
  c : PMIOPort  Port=3  Side=Right
  A : PMIOPort  Tag=PMCPort  Port=4  Side=Left
  B : PMIOPort  Tag=PMCPort  Port=5  Side=Left
  C : PMIOPort  Tag=PMCPort  Port=6  Side=Left
  Vc_abc : Outport  VectorParamsAs1DForOutWhenUnconnected=off
  Iinv_abc : Outport  Port=2  VectorParamsAs1DForOutWhenUnconnected=off
  wires:
  Three-Phase V-I Measurement/1 -> Vc_abc/1
  Three-Phase V-I Measurement/2 -> Iinv_abc/1
  connections:
  Three-Phase Series RLC Branch2/LConn3 -- Three-Phase V-I Measurement/RConn3 -- Three-Phase Transformer (Two Windings)/RConn3
  Three-Phase Series RLC Branch2/LConn2 -- Three-Phase V-I Measurement/RConn2 -- Three-Phase Transformer (Two Windings)/RConn2
  Three-Phase Series RLC Branch2/LConn1 -- Three-Phase V-I Measurement/RConn1 -- Three-Phase Transformer (Two Windings)/RConn1
  Three-Phase Series RLC Branch2/RConn2 -- Ground/LConn1 -- Three-Phase Series RLC Branch2/RConn3 -- Three-Phase Series RLC Branch2/RConn1
  A/RConn1 -- Li/RConn1
  B/RConn1 -- Li/RConn2
  Li/RConn3 -- C/RConn1
  Three-Phase V-I Measurement/LConn1 -- Li/LConn1
  Three-Phase V-I Measurement/LConn2 -- Li/LConn2
  Three-Phase V-I Measurement/LConn3 -- Li/LConn3
  a/RConn1 -- Three-Phase Transformer (Two Windings)/LConn1
  b/RConn1 -- Three-Phase Transformer (Two Windings)/LConn2
  c/RConn1 -- Three-Phase Transformer (Two Windings)/LConn3

== system Battery_Connected_3_Phase_GridTied_Inverter/Battery Connected 3 Phase Grid Tied Inverter/LPF ==
  Vc : Inport
  Iconv : Inport  Port=2
  Vo : Inport  Port=3
  Io : Inport  Port=4
  Vdc : Inport  Port=5
  Constant1 : Constant
  Constant3 : Constant
  LPF_abc : Subsystem
  LPF_abc1 : Subsystem
  LPF_abc2 : Subsystem
  LPF_abc3 : Subsystem
  Switch : Switch  Criteria=u2 > Threshold  Threshold=0.5  SaturateOnIntegerOverflow=off  InputSameDT=off
  Transport Delay : TransportDelay  DelayTime=tinit
  measurement_LPF : TransferFcn  Denominator=[a2_lpf a1_lpf 1]
  Vc_f : Outport  VectorParamsAs1DForOutWhenUnconnected=off
  Iconv_f : Outport  Port=2  VectorParamsAs1DForOutWhenUnconnected=off
  Vo_f : Outport  Port=3  VectorParamsAs1DForOutWhenUnconnected=off
  Io_f : Outport  Port=4  VectorParamsAs1DForOutWhenUnconnected=off
  Vdc_f : Outport  Port=5  VectorParamsAs1DForOutWhenUnconnected=off
  wires:
  Vc/1 -> LPF_abc/1(X)
  LPF_abc/1(X_f) -> Vc_f/1
  Iconv/1 -> LPF_abc1/1(X)
  LPF_abc1/1(X_f) -> Iconv_f/1
  Vo/1 -> LPF_abc2/1(X)
  LPF_abc2/1(X_f) -> Vo_f/1
  Io/1 -> LPF_abc3/1(X)
  LPF_abc3/1(X_f) -> Io_f/1
  Constant3/1 -> Transport Delay/1
  Transport Delay/1 -> Switch/2
  Constant1/1 -> Switch/3
  Vdc/1 -> measurement_LPF/1
  measurement_LPF/1 -> Switch/1
  Switch/1 -> Vdc_f/1

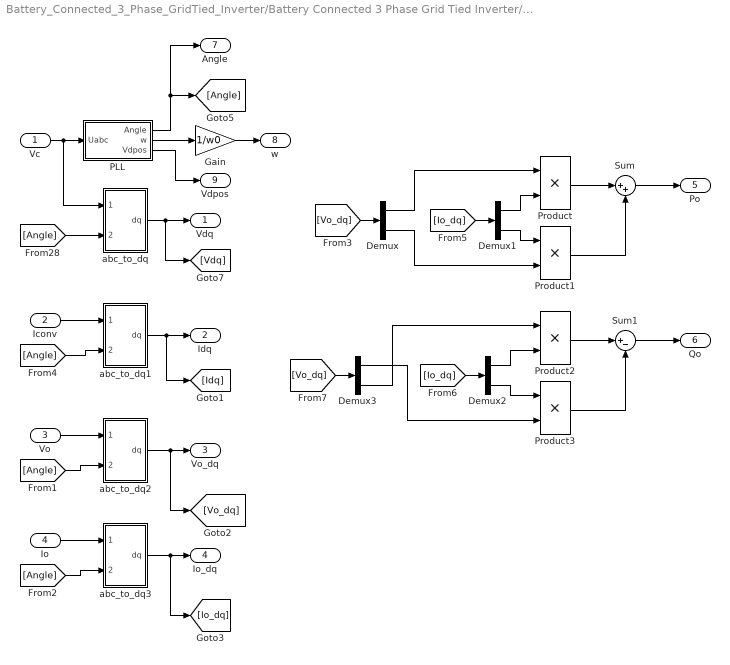
== system Battery_Connected_3_Phase_GridTied_Inverter/Battery Connected 3 Phase Grid Tied Inverter/Measurement ==
  Vc : Inport
  Iconv : Inport  Port=2
  Vo : Inport  Port=3
  Io : Inport  Port=4
  Demux{,1..3} (4 alike) : Demux  Outputs=2
  Gain : Gain  Gain=1/w0
  PLL : Subsystem
  Product{,1..3} (4 alike) : Product
  Sum : Sum  Inputs=|++
  Sum1 : Sum  Inputs=|+-
  abc_to_dq : Subsystem
  abc_to_dq1 : Subsystem
  abc_to_dq2 : Subsystem
  abc_to_dq3 : Subsystem
  Vdq : Outport  VectorParamsAs1DForOutWhenUnconnected=off
  Idq : Outport  Port=2  VectorParamsAs1DForOutWhenUnconnected=off
  Vo_dq : Outport  Port=3  VectorParamsAs1DForOutWhenUnconnected=off
  Io_dq : Outport  Port=4  VectorParamsAs1DForOutWhenUnconnected=off
  Po : Outport  Port=5  VectorParamsAs1DForOutWhenUnconnected=off
  Qo : Outport  Port=6  VectorParamsAs1DForOutWhenUnconnected=off
  Angle : Outport  Port=7  VectorParamsAs1DForOutWhenUnconnected=off
  w : Outport  Port=8  VectorParamsAs1DForOutWhenUnconnected=off
  Vdpos : Outport  Port=9  VectorParamsAs1DForOutWhenUnconnected=off
  wires:
  Demux/1 -> Product/1
  Product1/1 -> Sum/2
  Product/1 -> Sum/1
  Sum/1 -> Po/1
  Sum1/1 -> Qo/1
  Product2/1 -> Sum1/1
  Product3/1 -> Sum1/2
  Gain/1 -> w/1
  Vc/1 -> abc_to_dq/1(abc), PLL/1(Uabc)
  PLL/1(Angle) -> Angle/1, [Angle]
  PLL/2(w) -> Gain/1
  [Angle] -> abc_to_dq/2(theta)
  abc_to_dq/1(dq) -> [Vdq], Vdq/1
  Iconv/1 -> abc_to_dq1/1(abc)
  [Angle] -> abc_to_dq1/2(theta)
  abc_to_dq1/1(dq) -> [Idq], Idq/1
  Vo/1 -> abc_to_dq2/1(abc)
  abc_to_dq2/1(dq) -> [Vo_dq], Vo_dq/1
  [Angle] -> abc_to_dq2/2(theta)
  [Angle] -> abc_to_dq3/2(theta)
  abc_to_dq3/1(dq) -> [Io_dq], Io_dq/1
  Io/1 -> abc_to_dq3/1(abc)
  [Vo_dq] -> Demux/1
  [Io_dq] -> Demux1/1
  Demux1/1 -> Product/2
  Demux1/2 -> Product1/1
  Demux/2 -> Product1/2
  [Io_dq] -> Demux2/1
  Demux2/1 -> Product2/2
  Demux2/2 -> Product3/1
  [Vo_dq] -> Demux3/1
  Demux3/2 -> Product2/1
  Demux3/1 -> Product3/2
  PLL/3(Vdpos) -> Vdpos/1

== system Battery_Connected_3_Phase_GridTied_Inverter/Battery Connected 3 Phase Grid Tied Inverter/P_Control ==
  Pref : Inport
  P : Inport  Port=2
  Constant1 : Constant  Value=0
  Constant3 : Constant
  Pcontrol_PI : slpidlib/PID Controller  Controller=PI  Form=Parallel  TimeDomain=Continuous-time  UseExternalTs=off  SampleTime=-1  IntegratorMethod=Forward Euler  FilterMethod=Forward Euler  ControllerParametersSource=internal  P=Kpp  I=Kip  UseKiTs=off  D=0  N=100  UseFilter=on  TunerSelectOption=Transfer Function Based (PID Tuner App)  InitialConditionSource=internal  InitialConditionForIntegrator=Ia_init  InitialConditionForFilter=0  DifferentiatorICPrevScaledInput=0  ExternalReset=none  TrackingMode=off  Kt=1  LimitOutput=on  SatLimitsSource=internal  UpperSaturationLimit=Ia_limit  LowerSaturationLimit=0  LinearizeAsGain=on  AntiWindupMode=none  Kb=1  POutMin=[]  POutMax=[]  IOutMin=[]  IOutMax=[]  DOutMin=[]  DOutMax=[]  NOutMin=[]  NOutMax=[]  SumOutMin=[]  SumOutMax=[]  SaturationOutMin=[]  SaturationOutMax=[]  PParamMin=[]  PParamMax=[]  IParamMin=[]  IParamMax=[]  DParamMin=[]  DParamMax=[]  NParamMin=[]  NParamMax=[]  KbParamMin=[]  KbParamMax=[]  KtParamMin=[]  KtParamMax=[]  KbOutMin=[]  KbOutMax=[]  KtOutMin=[]  KtOutMax=[]  IntegratorOutMin=[]  IntegratorOutMax=[]  FilterOutMin=[]  FilterOutMax=[]  SumI1OutMin=[]  SumI1OutMax=[]  SumI2OutMin=[]  SumI2OutMax=[]  SumI3OutMin=[]  SumI3OutMax=[]  SumI4OutMin=[]  SumI4OutMax=[]  SumDOutMin=[]  SumDOutMax=[]  DifferentiatorOutMin=[]  DifferentiatorOutMax=[]  FilterDiffOutCoefMin=[]  FilterDiffOutCoefMax=[]  ReciprocalOutMin=[]  ReciprocalOutMax=[]  SumDenOutMin=[]  SumDenOutMax=[]  SumNumOutMin=[]  SumNumOutMax=[]  DivideOutMin=[]  DivideOutMax=[]  UdiffTsProdOutMin=[]  UdiffTsProdOutMax=[]  NTsProdOutMin=[]  NTsProdOutMax=[]  UintegralTsProdOutMin=[]  UintegralTsProdOutMax=[]  UngainTsProdOutMin=[]  UngainTsProdOutMax=[]  IntegratorContinuousStateAttributes=''  IntegratorStateMustResolveToSignalObject=off  IntegratorRTWStateStorageClass=Auto  FilterContinuousStateAttributes=''  FilterStateMustResolveToSignalObject=off  FilterRTWStateStorageClass=Auto  ParallelPVariant=InternalParameters  IdealPVariant=Disabled  IVariant=InternalParameters  DVariant=Disabled  IntegratorVariant=Continuous  SatVariant=Enabled  AWVariant=Passthrough  PCopyVariant=Disabled  TRVariant=Disabled  FdbkBlocksVariant=Forward  IdealPFdbkVariant=Disabled  SatFdbkVariant=Disabled  DerivativeFilterVariant=Disabled  NVariant=Disabled  NCopyVariant=Disabled_SignalSpec  FilterICVariant=Disabled  IntegratorICVariant=InternalICs  ExternalResetVariant=Disabled  TRSumVariant=Passthrough  SumFdbkVariant=Disabled  SumVariant=Sum_PI  TsampFilterVariant=InternalTs  TsampNgainVariant=Passthrough  TsampIntegralVariant=Passthrough  ExternalSaturationOutDataTypeStr=Inherit: Same as second input  aMode=0
  Sum3 : Sum  Inputs=|+-
  Switch : Switch  Criteria=u2 > Threshold  Threshold=0.5  SaturateOnIntegerOverflow=off  InputSameDT=off
  Transport Delay : TransportDelay  DelayTime=0.5
  Iact_ref : Outport  VectorParamsAs1DForOutWhenUnconnected=off
  wires:
  Pref/1 -> Sum3/1
  P/1 -> Sum3/2
  Pcontrol_PI/1 -> Iact_ref/1
  Sum3/1 -> Switch/1
  Constant1/1 -> Switch/3
  Constant3/1 -> Transport Delay/1
  Transport Delay/1 -> Switch/2
  Switch/1 -> Pcontrol_PI/1

== system Battery_Connected_3_Phase_GridTied_Inverter/Battery Connected 3 Phase Grid Tied Inverter/Psource ==
  Constant1 : Constant  Value=dP4
  Constant2 : Constant  Value=Pinit
  Constant3 : Constant  Value=dP2
  Constant4 : Constant  Value=dP1
  Constant5 : Constant  Value=dP3
  Gain : Gain  Gain=Sb
  Saturation : Saturate  UpperLimit=2  LowerLimit=0
  Sum1 : Sum  Inputs=+++++
  Transport Delay1 : TransportDelay  DelayTime=tP1
  Transport Delay2 : TransportDelay  DelayTime=tP4
  Transport Delay3 : TransportDelay  DelayTime=tP2
  Transport Delay4 : TransportDelay  DelayTime=tP3
  Psource : Outport  VectorParamsAs1DForOutWhenUnconnected=off
  wires:
  Constant2/1 -> Sum1/1
  Constant3/1 -> Transport Delay3/1
  Transport Delay3/1 -> Sum1/3
  Transport Delay4/1 -> Sum1/4
  Constant4/1 -> Transport Delay1/1
  Transport Delay1/1 -> Sum1/2
  Constant5/1 -> Transport Delay4/1
  Constant1/1 -> Transport Delay2/1
  Transport Delay2/1 -> Sum1/5
  Gain/1 -> Psource/1
  Sum1/1 -> Saturation/1
  Saturation/1 -> Gain/1

== system Battery_Connected_3_Phase_GridTied_Inverter/Battery Connected 3 Phase Grid Tied Inverter/Q_Control ==
  Qref : Inport
  Q : Inport  Port=2
  Qcontrol_PI1 : slpidlib/PID Controller  Controller=PI  Form=Parallel  TimeDomain=Continuous-time  UseExternalTs=off  SampleTime=-1  IntegratorMethod=Forward Euler  FilterMethod=Forward Euler  ControllerParametersSource=internal  P=Kpq  I=Kiq  UseKiTs=off  D=0  N=100  UseFilter=on  TunerSelectOption=Transfer Function Based (PID Tuner App)  InitialConditionSource=internal  InitialConditionForIntegrator=Ir_init  InitialConditionForFilter=0  DifferentiatorICPrevScaledInput=0  ExternalReset=none  TrackingMode=off  Kt=1  LimitOutput=on  SatLimitsSource=internal  UpperSaturationLimit=Ir_limit  LowerSaturationLimit=-Ir_limit  LinearizeAsGain=on  AntiWindupMode=clamping  Kb=1  POutMin=[]  POutMax=[]  IOutMin=[]  IOutMax=[]  DOutMin=[]  DOutMax=[]  NOutMin=[]  NOutMax=[]  SumOutMin=[]  SumOutMax=[]  SaturationOutMin=[]  SaturationOutMax=[]  PParamMin=[]  PParamMax=[]  IParamMin=[]  IParamMax=[]  DParamMin=[]  DParamMax=[]  NParamMin=[]  NParamMax=[]  KbParamMin=[]  KbParamMax=[]  KtParamMin=[]  KtParamMax=[]  KbOutMin=[]  KbOutMax=[]  KtOutMin=[]  KtOutMax=[]  IntegratorOutMin=[]  IntegratorOutMax=[]  FilterOutMin=[]  FilterOutMax=[]  SumI1OutMin=[]  SumI1OutMax=[]  SumI2OutMin=[]  SumI2OutMax=[]  SumI3OutMin=[]  SumI3OutMax=[]  SumI4OutMin=[]  SumI4OutMax=[]  SumDOutMin=[]  SumDOutMax=[]  DifferentiatorOutMin=[]  DifferentiatorOutMax=[]  FilterDiffOutCoefMin=[]  FilterDiffOutCoefMax=[]  ReciprocalOutMin=[]  ReciprocalOutMax=[]  SumDenOutMin=[]  SumDenOutMax=[]  SumNumOutMin=[]  SumNumOutMax=[]  DivideOutMin=[]  DivideOutMax=[]  UdiffTsProdOutMin=[]  UdiffTsProdOutMax=[]  NTsProdOutMin=[]  NTsProdOutMax=[]  UintegralTsProdOutMin=[]  UintegralTsProdOutMax=[]  UngainTsProdOutMin=[]  UngainTsProdOutMax=[]  IntegratorContinuousStateAttributes=''  IntegratorStateMustResolveToSignalObject=off  IntegratorRTWStateStorageClass=Auto  FilterContinuousStateAttributes=''  FilterStateMustResolveToSignalObject=off  FilterRTWStateStorageClass=Auto  ParallelPVariant=InternalParameters  IdealPVariant=Disabled  IVariant=InternalParameters  DVariant=Disabled  IntegratorVariant=Continuous  SatVariant=Enabled  AWVariant=ContClampingParallel  PCopyVariant=Disabled  TRVariant=Disabled  FdbkBlocksVariant=Forward  IdealPFdbkVariant=Disabled  SatFdbkVariant=Disabled  DerivativeFilterVariant=Disabled  NVariant=Disabled  NCopyVariant=Disabled_SignalSpec  FilterICVariant=Disabled  IntegratorICVariant=InternalICs  ExternalResetVariant=Disabled  TRSumVariant=Passthrough  SumFdbkVariant=Disabled  SumVariant=Sum_PI  TsampFilterVariant=InternalTs  TsampNgainVariant=Passthrough  TsampIntegralVariant=Passthrough  ExternalSaturationOutDataTypeStr=Inherit: Same as second input  aMode=0
  Sum3 : Sum  Inputs=|+-
  Ireact_ref : Outport  VectorParamsAs1DForOutWhenUnconnected=off
  wires:
  Qref/1 -> Sum3/1
  Sum3/1 -> Qcontrol_PI1/1
  Qcontrol_PI1/1 -> Ireact_ref/1
  Q/1 -> Sum3/2
